simulink model "pi_button"  (R2017a)
settings: Solver=VariableStepAuto  StartTime=0.0  StopTime=inf  RelTol=1e-3
undefined symbols (not defined in the file or in its folder): Green, led0
libraries: embdlinuxlib x3
settings Model: SimulationMode=external  Creator=WARA  LastModifiedBy=Vincent

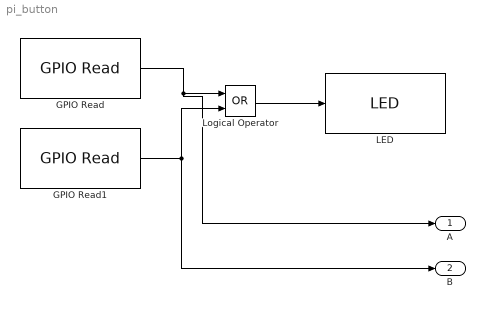
== system pi_button ==
  GPIO Read : embdlinuxlib/GPIO Read  board=Pi 3 Model B  gpio=22  internalResistor=Off  sampleTime=0.1  direction=Input  blockPlatform=Raspberry Pi
  GPIO Read1 : embdlinuxlib/GPIO Read  board=Pi 3 Model B  gpio=27  internalResistor=Off  sampleTime=0.1  direction=Input  blockPlatform=Raspberry Pi
  LED : embdlinuxlib/LED  board=Pi 2 Model B  led=led0 (Green)  blockPlatform=Raspberry Pi
  Logical Operator : Logic  Operator=OR  AllPortsSameDT=off  OutDataTypeStr=boolean
  A : Outport
  B : Outport  Port=2
  wires:
  Logical Operator/1 -> LED/1
  GPIO Read/1 -> A/1, Logical Operator/1
  GPIO Read1/1 -> B/1, Logical Operator/2
